simulink model "PID_28Nov_Mod"  (R2021b)
settings: Solver=VariableStepAuto  StartTime=0.0  StopTime=10.0  RelTol=1e-3
values from neighbouring files (symbols this model uses):
  Kp = 450    [CC_PID.mat]
  set_spd = 50    [CC_PID.mat]
undefined symbols (not defined in the file or in its folder): DiscIntNeverNeededParam
libraries: simulink x1
settings Model: Creator=Manmath Kharade  LastModifiedBy=Manmath Kharade

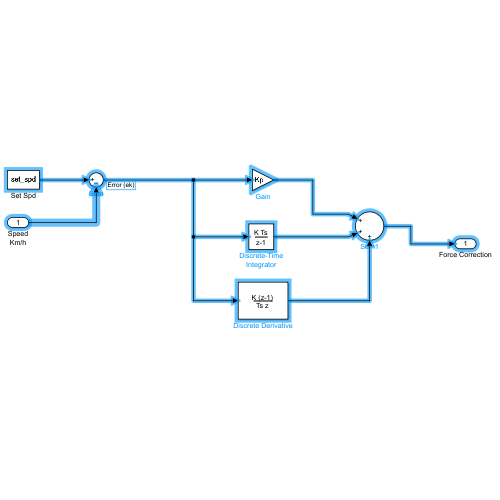
[thumbnail: Simulink's stored preview of the top-level diagram]
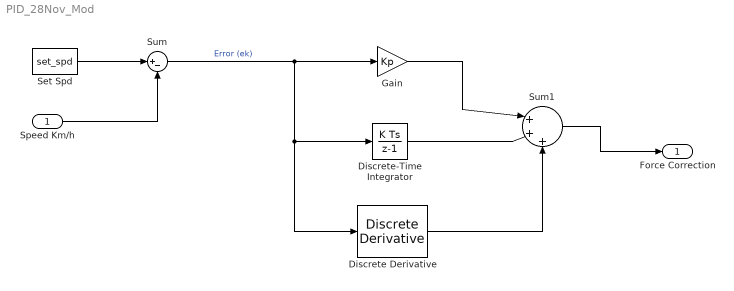
== system PID_28Nov_Mod ==
  Speed Km/h : Inport
  Discrete Derivative : simulink/Discrete/Discrete Derivative  gainval=Kd  ICPrevScaledInput=0.0  OutMin=[]  OutMax=[]  OutDataType=fixdt(1, 16)  OutScaling=2^-10  DoSatur=off
  Discrete-Time Integrator : DiscreteIntegrator  gainval=Ki  SampleTime=0.01  ICPrevOutput=DiscIntNeverNeededParam  ICPrevScaledInput=DiscIntNeverNeededParam
  Gain : Gain  Gain=Kp
  Set Spd : Constant  Value=set_spd
  Sum : Sum  Inputs=|+-
  Sum1 : Sum  Inputs=|+++
  Force Correction : Outport
  wires:
  Discrete Derivative/1 -> Sum1/3
  Sum/1 -> Gain/1, Discrete Derivative/1, Discrete-Time Integrator/1  "Error (ek)"
  Gain/1 -> Sum1/1
  Discrete-Time Integrator/1 -> Sum1/2
  Set Spd/1 -> Sum/1
  Sum1/1 -> Force Correction/1
  Speed Km/h/1 -> Sum/2
